simulink model "Elc343_Term_Project_Simulink"  (R2015b)
settings: Solver=VariableStepAuto  StartTime=0.0  StopTime=10.0  RelTol=1e-3
undefined symbols (not defined in the file): a, b
settings Model: Creator=bryanguner  LastModifiedBy=bryanguner

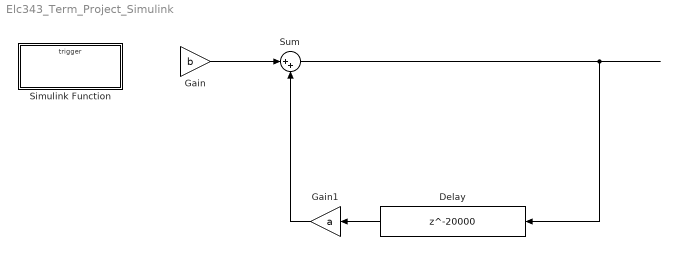
== system Elc343_Term_Project_Simulink ==
  Delay : Delay  DelayLength=20000
  Gain : Gain  Gain=b
  Gain1 : Gain  Gain=a
  Simulink Function : Subsystem  TreatAsAtomicUnit=on
  Sum : Sum  Inputs=|++
  wires:
  Gain/1 -> Sum/1
  Gain1/1 -> Sum/2
  Delay/1 -> Gain1/1
  Sum/1 -> Delay/1

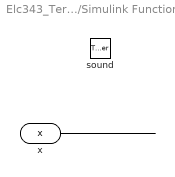
== system Elc343_Term_Project_Simulink/Simulink Function ==
  sound : TriggerPort  TriggerType=function-call  IsSimulinkFunction=on  FunctionName=sound
  x : ArgIn  DisableCoverage=on  ArgumentName=x
  wires:
  x/1 -> ?
